simulink model "APT"  (R2019a)
settings: Solver=FixedStepDiscrete  StartTime=0.0  StopTime=stop_time  RelTol=1e-3
InitFcn:
  | APT_callback_init
StopFcn:
  | APT_callback_stop
undefined symbols (not defined in the file): Ts_system
libraries: simulink x3
settings Model: Creator=Ross  LastModifiedBy=Ross
settings DataIOCC: ReturnWorkspaceOutputs=off
settings OptimizationCC: BlockReduction=off  ConditionallyExecuteInputs=off  DefaultParameterBehavior=Inlined
settings DebuggingCC: ReadBeforeWriteMsg=DisableAll  WriteAfterWriteMsg=DisableAll  WriteAfterReadMsg=DisableAll  AlgebraicLoopMsg=error  MultiTaskDSMMsg=none  SingleTaskRateTransMsg=error  PregeneratedLibrarySubsystemCodeDiagnostic=none  ArithmeticOperatorsInVariantConditions=warning
settings HardwareCC: ProdBitPerPointer=32  ProdBitPerSizeT=32  ProdBitPerPtrDiffT=32  ProdLargestAtomicFloat=None  ProdIntDivRoundTo=Undefined  ProdEndianess=Unspecified  ProdWordSize=32  ProdHWDeviceType=ASIC/FPGA->ASIC/FPGA  TargetBitPerPointer=64  TargetBitPerSizeT=64  TargetBitPerPtrDiffT=64  TargetLongLongMode=on  TargetIntDivRoundTo=Zero  TargetEndianess=LittleEndian  TargetWordSize=64  TargetHWDeviceType=Custom Processor->MATLAB Host Computer  ProdEqTarget=off
settings ModelReferenceCC: UpdateModelReferenceTargets=IfOutOfDate
settings SFSimCC: SFSimEcho=off  SimUseLocalCustomCode=off
settings RTWCC: RTWUseLocalCustomCode=off

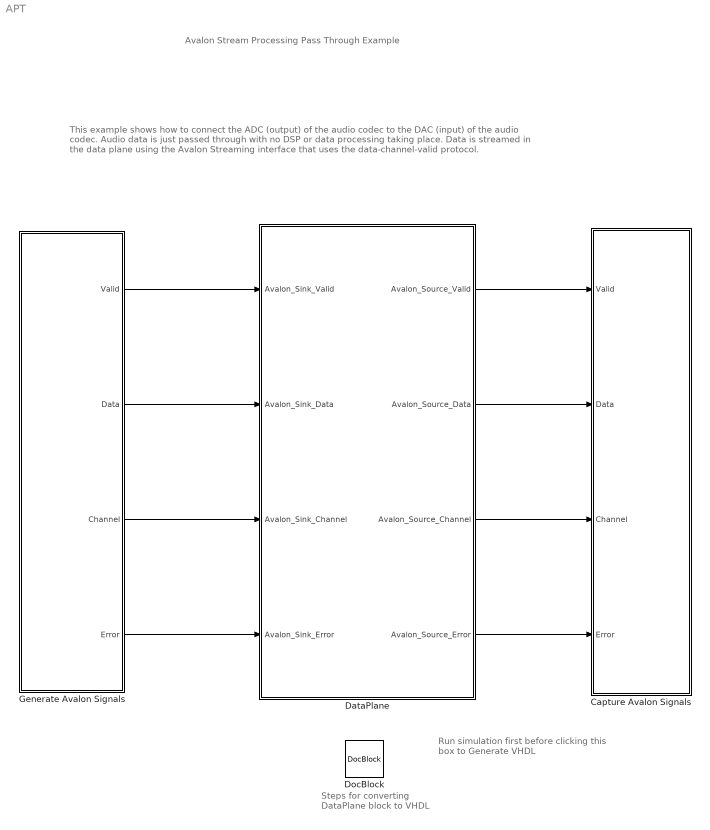
== system APT ==
  note: Run simulation first
      | before clicking this box to
      | Generate VHDL
  note: This example shows how to connect the ADC (output) of the audio codec to the DAC (input) of the audio codec. Audio data is just passed through with no DSP or data processing taking place. Data is streamed in the data plane using the Avalon Streaming interface that uses the data-channel-valid protocol.
  note: Steps for converting
      | DataPlane block
      | to VHDL
  note: Avalon Stream Processing
      | Pass Through Example
  Capture Avalon Signals : Subsystem
  DataPlane : Subsystem  TreatAsAtomicUnit=on
  DocBlock : simulink/Model-Wide Utilities/DocBlock  DocumentType=HTML
  Generate Avalon Signals : Subsystem
  wires:
  Generate Avalon Signals/2(Data) -> DataPlane/2(Avalon_Sink_Data)
  Generate Avalon Signals/1(Valid) -> DataPlane/1(Avalon_Sink_Valid)
  Generate Avalon Signals/3(Channel) -> DataPlane/3(Avalon_Sink_Channel)
  Generate Avalon Signals/4(Error) -> DataPlane/4(Avalon_Sink_Error)
  DataPlane/2(Avalon_Source_Data) -> Capture Avalon Signals/2(Data)
  DataPlane/1(Avalon_Source_Valid) -> Capture Avalon Signals/1(Valid)
  DataPlane/3(Avalon_Source_Channel) -> Capture Avalon Signals/3(Channel)
  DataPlane/4(Avalon_Source_Error) -> Capture Avalon Signals/4(Error)

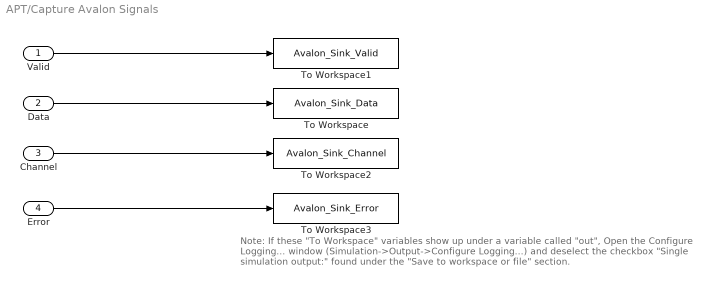
== system APT/Capture Avalon Signals ==
  note: Note:  If these "To Workspace" variables show up under a variable called "out",
      | Open the Configure Logging... window (Simulation->Output->Configure Logging...)
      | and deselect the checkbox "Single simulation output:" found under the "Save to workspace or file" section.
  Valid : Inport
  Data : Inport  Port=2
  Channel : Inport  Port=3
  Error : Inport  Port=4
  To Workspace : ToWorkspace  VariableName=Avalon_Sink_Data  SaveFormat=Timeseries  SampleTime=-1
  To Workspace1 : ToWorkspace  VariableName=Avalon_Sink_Valid  SaveFormat=Timeseries  SampleTime=-1
  To Workspace2 : ToWorkspace  VariableName=Avalon_Sink_Channel  SaveFormat=Timeseries  SampleTime=-1
  To Workspace3 : ToWorkspace  VariableName=Avalon_Sink_Error  SaveFormat=Timeseries  SampleTime=-1
  wires:
  Data/1 -> To Workspace/1
  Valid/1 -> To Workspace1/1
  Error/1 -> To Workspace3/1
  Channel/1 -> To Workspace2/1

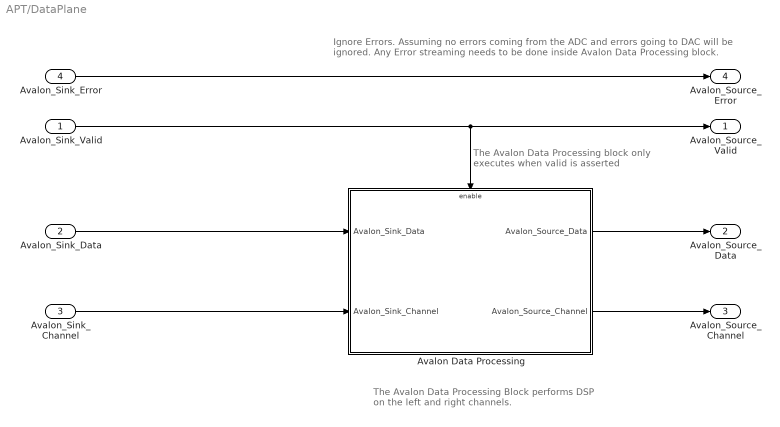
== system APT/DataPlane ==
  note: The Avalon Data Processing Block
      | performs DSP on the left and right channels.
  note: The Avalon Data Processing block
      | only executes when valid is asserted
  note: Ignore Errors.
      | Assuming no errors coming from the ADC and errors going to DAC will be ignored.
      | Any Error streaming needs to be done inside Avalon Data Processing block.
  Avalon_Sink_Valid : Inport
  Avalon_Sink_Data : Inport  Port=2
  Avalon_Sink_Channel : Inport  Port=3
  Avalon_Sink_Error : Inport  Port=4
  Avalon Data Processing : Subsystem  TreatAsAtomicUnit=on
  Avalon_Source_Valid : Outport
  Avalon_Source_Data : Outport  Port=2
  Avalon_Source_Channel : Outport  Port=3
  Avalon_Source_Error : Outport  Port=4
  wires:
  Avalon_Sink_Channel/1 -> Avalon Data Processing/2(Avalon_Sink_Channel)
  Avalon_Sink_Error/1 -> Avalon_Source_Error/1
  Avalon Data Processing/1(Avalon_Source_Data) -> Avalon_Source_Data/1
  Avalon_Sink_Valid/1 -> Avalon Data Processing/Enable, Avalon_Source_Valid/1
  Avalon_Sink_Data/1 -> Avalon Data Processing/1(Avalon_Sink_Data)
  Avalon Data Processing/2(Avalon_Source_Channel) -> Avalon_Source_Channel/1

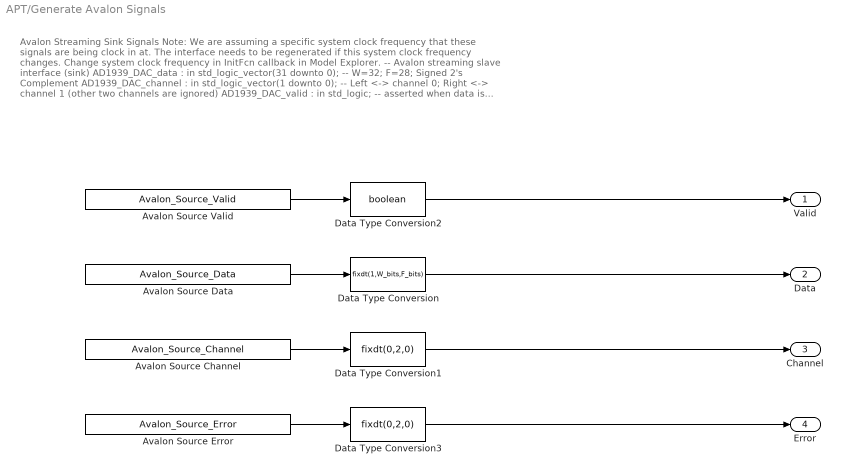
== system APT/Generate Avalon Signals ==
  note: Avalon Streaming Sink Signals
      | Note: We are assuming a specific system clock frequency that these signals are being clock in at.
      | The interface needs to be regenerated if this system clock frequency changes. Change system clock frequency in InitFcn callback in Model Explorer.
      |
      | -- Avalon streaming slave interface (sink)
      | AD1939_DAC_data : in std_logic_vector(31 downto 0); -- W=32; F=28; Signed 2's Complement
      | AD1939_DAC_channel : in std_logic_vector(1 downto 0); -- Left <-> channel 0; Right <-> channel 1 (other two channels are ignored)
      | AD1939_DAC_valid : in std_logic; -- asserted when data is valid
      | AD1939_DAC_error : in std_logic_vector(1 downto 0) -- error channel is ignored, assumed to be error free at this point
      |
      | For more information on the data-channel-valid protocol, s ee chapter 5 in Intel's Avalon Interfaced Specification (p. 40) at https://www.intel.com/content/dam/www/programmable/us/en/pdfs/literature/manual/mnl_avalon_spec.pdf
  Avalon Source Channel : FromWorkspace  VariableName=Avalon_Source_Channel  OutDataTypeStr=double  SampleTime=Ts_system
  "Avalon Source Data " : FromWorkspace  VariableName=Avalon_Source_Data  OutDataTypeStr=double  SampleTime=Ts_system
  Avalon Source Error : FromWorkspace  VariableName=Avalon_Source_Error  OutDataTypeStr=double  SampleTime=Ts_system
  Avalon Source Valid : FromWorkspace  VariableName=Avalon_Source_Valid  OutDataTypeStr=double  SampleTime=Ts_system
  Data Type Conversion : DataTypeConversion  OutDataTypeStr=fixdt(1,W_bits,F_bits)
  Data Type Conversion1 : DataTypeConversion  OutDataTypeStr=fixdt(0,2,0)
  Data Type Conversion2 : DataTypeConversion  OutDataTypeStr=boolean
  Data Type Conversion3 : DataTypeConversion  OutDataTypeStr=fixdt(0,2,0)
  Valid : Outport
  Data : Outport  Port=2
  Channel : Outport  Port=3
  Error : Outport  Port=4
  wires:
  Data Type Conversion1/1 -> Channel/1
  Data Type Conversion2/1 -> Valid/1
  Avalon Source Error/1 -> Data Type Conversion3/1
  Data Type Conversion/1 -> Data/1
  Avalon Source Valid/1 -> Data Type Conversion2/1
  Data Type Conversion3/1 -> Error/1
  Avalon Source Channel/1 -> Data Type Conversion1/1
  "Avalon Source Data "/1 -> Data Type Conversion/1

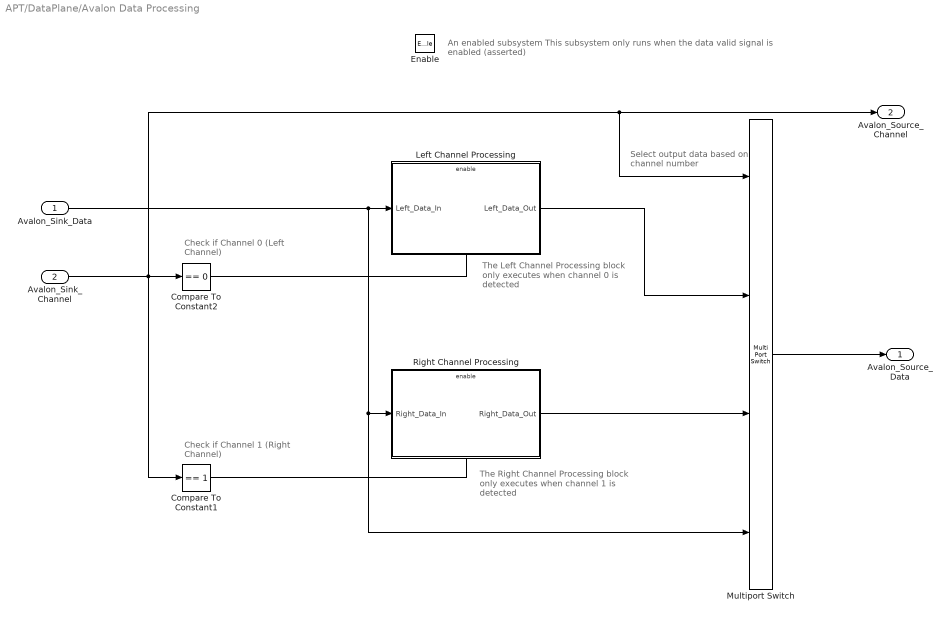
== system APT/DataPlane/Avalon Data Processing ==
  note: Select output data
      | based on channel number
  note: Check if Channel 0
      | (Left Channel)
  note: The Left Channel Processing block
      | only executes when channel 0
      | is detected
  note: The Right Channel Processing block
      | only executes when channel 1
      | is detected
  note: Check if Channel 1
      | (Right Channel)
  note: An enabled subsystem
      | This subsystem only runs when the data valid signal is enabled (asserted)
  Avalon_Sink_Data : Inport
  Avalon_Sink_Channel : Inport  Port=2
  Enable : EnablePort
  Compare To Constant1 : simulink/Logic and Bit Operations/Compare To Constant  relop===  const=1  OutDataTypeStr=boolean
  Compare To Constant2 : simulink/Logic and Bit Operations/Compare To Constant  relop===  const=0  OutDataTypeStr=boolean
  Left Channel Processing : Subsystem  TreatAsAtomicUnit=on
  Multiport Switch : MultiPortSwitch  DataPortOrder=Zero-based contiguous  zeroidx=on
  Right Channel Processing : Subsystem  TreatAsAtomicUnit=on
  Avalon_Source_Data : Outport  InitialOutput=0
  Avalon_Source_Channel : Outport  Port=2  InitialOutput=0
  wires:
  Avalon_Sink_Channel/1 -> Avalon_Source_Channel/1, Multiport Switch/1, Compare To Constant1/1, Compare To Constant2/1
  Compare To Constant2/1 -> Left Channel Processing/Enable
  Compare To Constant1/1 -> Right Channel Processing/Enable
  Avalon_Sink_Data/1 -> Multiport Switch/4, Right Channel Processing/1(Right_Data_In), Left Channel Processing/1(Left_Data_In)
  Left Channel Processing/1("Left_Data_Out ") -> Multiport Switch/2
  Right Channel Processing/1("Right_Data_Out ") -> Multiport Switch/3
  Multiport Switch/1 -> Avalon_Source_Data/1

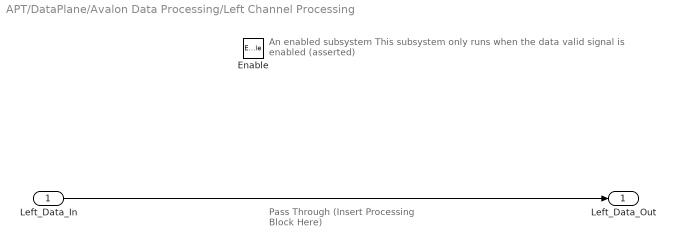
== system APT/DataPlane/Avalon Data Processing/Left Channel Processing ==
  note: Pass Through
      | (Insert Processing Block Here)
  note: An enabled subsystem
      | This subsystem only runs when the data valid signal is enabled (asserted)
  Left_Data_In : Inport
  Enable : EnablePort
  "Left_Data_Out " : Outport  InitialOutput=0
  wires:
  Left_Data_In/1 -> "Left_Data_Out "/1

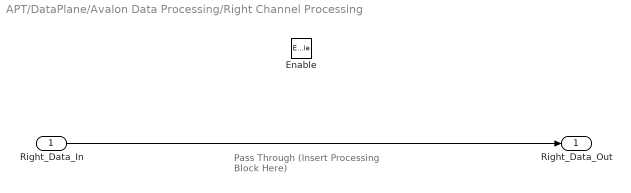
== system APT/DataPlane/Avalon Data Processing/Right Channel Processing ==
  note: Pass Through
      | (Insert Processing Block Here)
  Right_Data_In : Inport
  Enable : EnablePort
  "Right_Data_Out " : Outport  InitialOutput=0
  wires:
  Right_Data_In/1 -> "Right_Data_Out "/1
